simulink model "sim_main_x12px23"  (R2014b)
settings: Solver=ode4  StartTime=0.0  StopTime=tof  FixedStep=dtSim  RelTol=1e-3
values from neighbouring files (symbols this model uses):
  alpha = 1    [main_pqr.m]    (also in main_x12px2.m = -1)
  Ar = -5    [main_pqr.m]    (also in main_x12px2.m = Arv(i))
  Arm1 = Arm1 + [0 a*max(abs(rData(:,3))) ; b*max(abs(rData(:,3))) 0]    [main_pqr.m]    (also in main_x12px2.m = -2)
  dtController = dtSim    (= 0.01)    [main_pqr.m]    (also in main_x12px2.m = 0.001)
  epsilon = 0.1    [main_pqr.m]    (also in main_x12px2.m)
  intLimit = 10    [main_pqr.m]    (also in main_x12px2.m)
  K2 = -2    [main_pqr.m]    (also in main_x12px2.m = -10)
  r0 = [0 0]'    [main_pqr.m]    (also in main_x12px2.m = 0)
  rmax = 10000    [main_pqr.m]    (also in main_x12px2.m)
  rmin = -rmax    (= -10000)    [main_pqr.m]    (also in main_x12px2.m)
  x0 = 1*x0    [main_pqr.m]    (also in main_x12px2.m = 10*x0)
settings Model: Creator=Alp  LastModifiedBy=alpmarangoz
settings SolverCC: AutoInsertRateTranBlk=on
settings DataIOCC: SignalLoggingSaveFormat=ModelDataLogs
settings OptimizationCC: ExpressionDepthLimit=2147483647
settings DebuggingCC: UnderspecifiedInitializationDetection=Classic  MergeDetectMultiDrivingBlocksExec=none  FcnCallInpInsideContextMsg=UseLocalSettings  StateNameClashWarn=warning
settings GRTTargetCC: CombineOutputUpdateFcns=off  GRTInterface=on

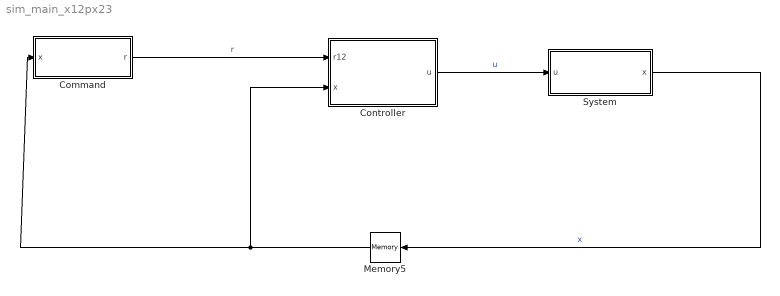
== system sim_main_x12px23 ==
  Command : Subsystem  TreatAsAtomicUnit=on  SystemSampleTime=dtController
  Controller : Subsystem  TreatAsAtomicUnit=on  SystemSampleTime=dtController
  Memory5 : Memory  X0=x0  InheritSampleTime=on  LinearizeMemory=on  LinearizeAsDelay=on
  System : Subsystem  TreatAsAtomicUnit=on
  wires:
  Command/1(r) -> Controller/1(r12)  "r"
  Controller/1(u) -> System/1(u)  "u"
  System/1(x) -> Memory5/1  "x"
  Memory5/1 -> Controller/2(x), Command/1(x)

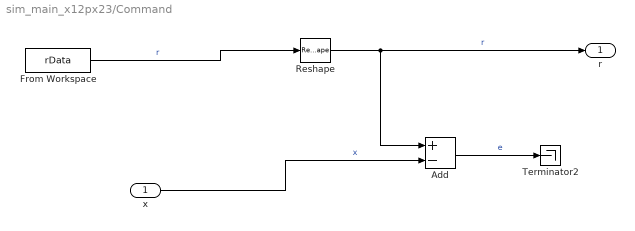
== system sim_main_x12px23/Command ==
  x : Inport
  Add : Sum  Inputs=+-
  From Workspace : FromWorkspace  VariableName=rData  OutputAfterFinalValue=Setting to zero
  Reshape : Reshape  OutputDimensionality=Column vector (2-D)
  Terminator2 : Terminator
  r : Outport
  wires:
  From Workspace/1 -> Reshape/1  "r"
  Reshape/1 -> r/1, Add/1  "r"
  x/1 -> Add/2  "x"
  Add/1 -> Terminator2/1  "e"

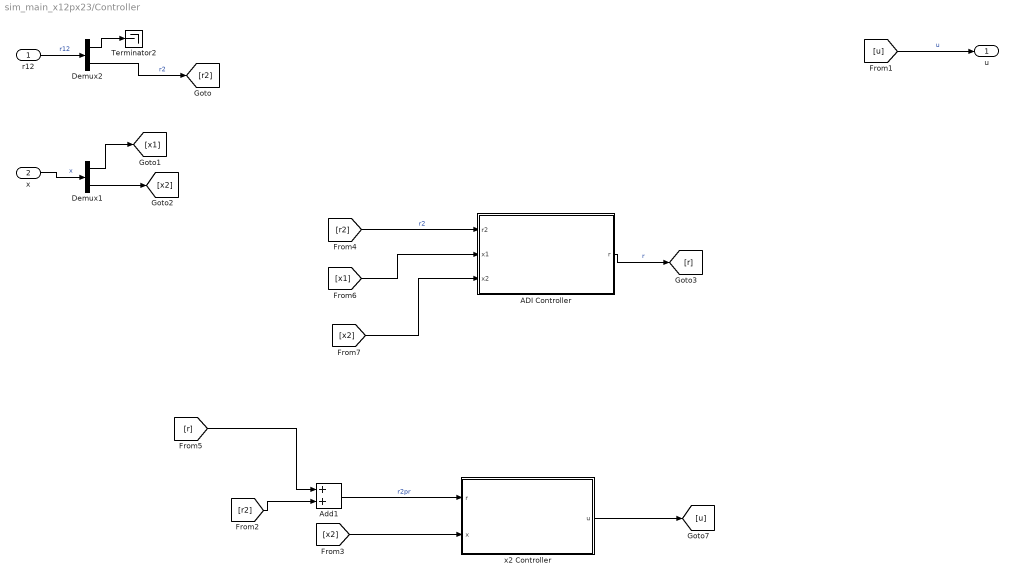
== system sim_main_x12px23/Controller ==
  r12 : Inport
  x : Inport  Port=2
  ADI Controller : Subsystem  TreatAsAtomicUnit=on
  Add1 : Sum
  Demux1 : Demux  Outputs=2
  Demux2 : Demux  Outputs=2
  Terminator2 : Terminator
  x2 Controller : Subsystem  TreatAsAtomicUnit=on
  u : Outport
  wires:
  [u] -> u/1  "u"
  Demux2/2 -> [r2]  "r2"
  Demux2/1 -> Terminator2/1
  r12/1 -> Demux2/1  "r12"
  x/1 -> Demux1/1  "x"
  Demux1/2 -> [x2]
  Demux1/1 -> [x1]
  [x2] -> x2 Controller/2(x)
  ADI Controller/1(r) -> [r]  "r"
  [r] -> Add1/1
  [r2] -> Add1/2
  Add1/1 -> x2 Controller/1(r)  "r2pr"
  [r2] -> ADI Controller/1(r2)  "r2"
  [x1] -> ADI Controller/2(x1)
  [x2] -> ADI Controller/3(x2)
  x2 Controller/1(u) -> [u]

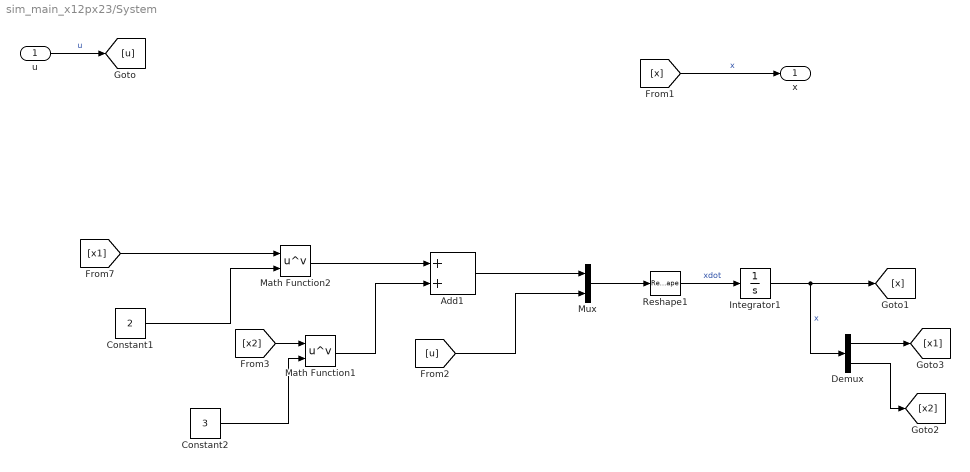
== system sim_main_x12px23/System ==
  u : Inport
  Add1 : Sum
  Constant1 : Constant  Value=2
  Constant2 : Constant  Value=3
  Demux : Demux  Outputs=2
  Integrator1 : Integrator  InitialCondition=x0  LimitOutput=on  UpperSaturationLimit=intLimit  LowerSaturationLimit=-intLimit
  Math Function1 : Math  Operator=pow  SaturateOnIntegerOverflow=on
  Math Function2 : Math  Operator=pow  SaturateOnIntegerOverflow=on
  Mux : Mux  Inputs=2
  Reshape1 : Reshape  OutputDimensionality=Column vector (2-D)
  x : Outport
  wires:
  u/1 -> [u]  "u"
  [x] -> x/1  "x"
  Reshape1/1 -> Integrator1/1  "xdot"
  Integrator1/1 -> [x], Demux/1  "x"
  Demux/2 -> [x2]
  Demux/1 -> [x1]
  [x1] -> Math Function2/1
  Constant1/1 -> Math Function2/2
  Math Function2/1 -> Add1/1
  Mux/1 -> Reshape1/1
  Add1/1 -> Mux/1
  [u] -> Mux/2
  [x2] -> Math Function1/1
  Math Function1/1 -> Add1/2
  Constant2/1 -> Math Function1/2

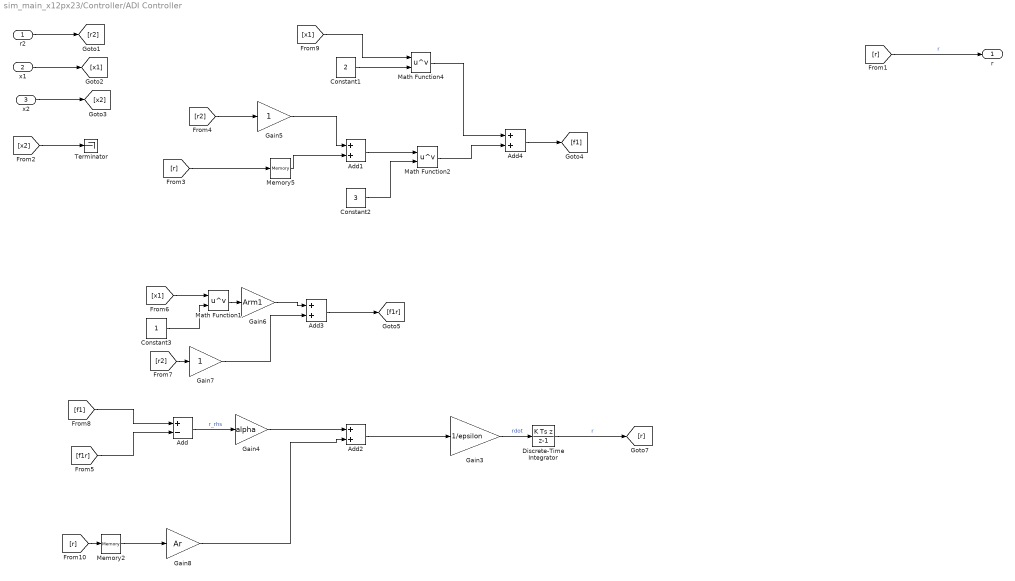
== system sim_main_x12px23/Controller/ADI Controller ==
  r2 : Inport
  x1 : Inport  Port=2
  x2 : Inport  Port=3
  Add : Sum  Inputs=+-
  Add{1..4} (4 alike) : Sum
  Constant1 : Constant  Value=2
  Constant2 : Constant  Value=3
  Constant3 : Constant
  Discrete-Time Integrator : DiscreteIntegrator  IntegratorMethod=Integration: Backward Euler  InitialCondition=r0  InitialConditionSetting=State (most efficient)  SampleTime=-1  LimitOutput=on  UpperSaturationLimit=rmax  LowerSaturationLimit=rmin
  Gain3 : Gain  Gain=1/epsilon
  Gain4 : Gain  Gain=alpha
  Gain5 : Gain
  Gain6 : Gain  Gain=Arm1
  Gain7 : Gain
  Gain8 : Gain  Gain=Ar
  Math Function1 : Math  Operator=pow  SaturateOnIntegerOverflow=on
  Math Function2 : Math  Operator=pow  SaturateOnIntegerOverflow=on
  Math Function4 : Math  Operator=pow  SaturateOnIntegerOverflow=on
  Memory2 : Memory  X0=r0  InheritSampleTime=on  LinearizeMemory=on  LinearizeAsDelay=on
  Memory5 : Memory  X0=r0  InheritSampleTime=on  LinearizeMemory=on  LinearizeAsDelay=on
  Terminator : Terminator
  r : Outport
  wires:
  Gain3/1 -> Discrete-Time Integrator/1  "rdot"
  Discrete-Time Integrator/1 -> [r]  "r"
  r2/1 -> [r2]
  x1/1 -> [x1]
  [r] -> r/1  "r"
  Add/1 -> Gain4/1  "r_rhs"
  [r] -> Memory5/1
  Memory5/1 -> Add1/2
  Gain5/1 -> Add1/1
  x2/1 -> [x2]
  [x2] -> Terminator/1
  Math Function1/1 -> Gain6/1
  [x1] -> Math Function1/1
  Constant3/1 -> Math Function1/2
  Gain6/1 -> Add3/1
  [r2] -> Gain7/1
  Add3/1 -> [f1r]
  Gain7/1 -> Add3/2
  [f1] -> Add/1
  [f1r] -> Add/2
  [r2] -> Gain5/1
  Gain4/1 -> Add2/1
  Add2/1 -> Gain3/1
  [r] -> Memory2/1
  Add4/1 -> [f1]
  Memory2/1 -> Gain8/1
  Gain8/1 -> Add2/2
  [x1] -> Math Function4/1
  Constant1/1 -> Math Function4/2
  Math Function4/1 -> Add4/1
  Math Function2/1 -> Add4/2
  Add1/1 -> Math Function2/1
  Constant2/1 -> Math Function2/2

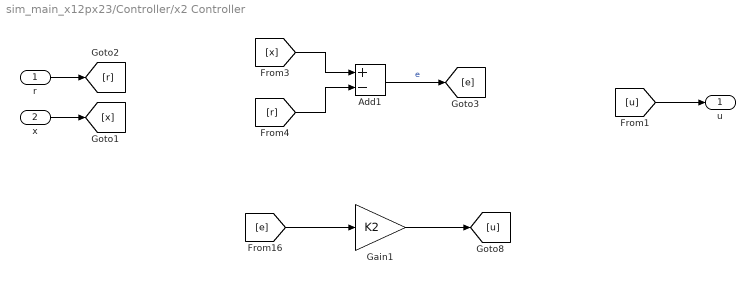
== system sim_main_x12px23/Controller/x2 Controller ==
  r : Inport
  x : Inport  Port=2
  Add1 : Sum  Inputs=+-
  Gain1 : Gain  Gain=K2
  u : Outport
  wires:
  [x] -> Add1/1
  [r] -> Add1/2
  Add1/1 -> [e]  "e"
  r/1 -> [r]
  x/1 -> [x]
  [u] -> u/1
  [e] -> Gain1/1
  Gain1/1 -> [u]
